simulink model "motor-DC-simulation"  (R2021b)
settings: Solver=VariableStepAuto  StartTime=0.0  StopTime=4  RelTol=1e-3
settings Model: Creator=nima8  LastModifiedBy=nima8

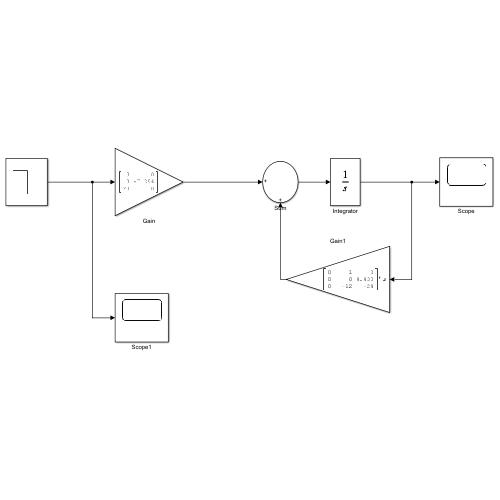
[thumbnail: Simulink's stored preview of the top-level diagram]
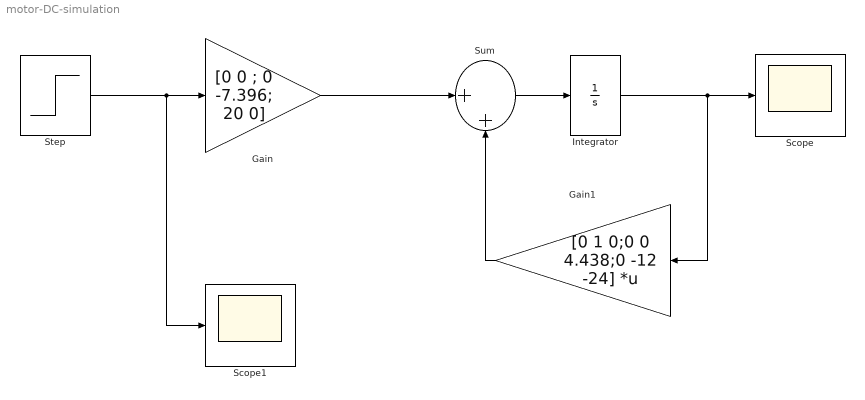
== system motor-DC-simulation ==
  Gain : Gain  Gain=[0 0 ; 0 -7.396; 20 0]
  Gain1 : Gain  Gain=[0 1 0;0 0 4.438;0 -12 -24]  Multiplication=Matrix(K*u)
  Integrator : Integrator  InitialCondition=[0 0 0;0 0 0]'
  Scope : Scope
  Scope1 : Scope
  Step : Step  Time=2  Before=3  After=-3  SampleTime=0
  Sum : Sum  Inputs=|++
  wires:
  Step/1 -> Scope1/1, Gain/1
  Gain/1 -> Sum/1
  Sum/1 -> Integrator/1
  Integrator/1 -> Scope/1, Gain1/1
  Gain1/1 -> Sum/2
